simulink model "Eq_Zeq_denominator"  (R2022a)
settings: Solver=VariableStepAuto  StartTime=0.0  StopTime=10.0  RelTol=1e-3
settings Model: Creator=umber  LastModifiedBy=umber

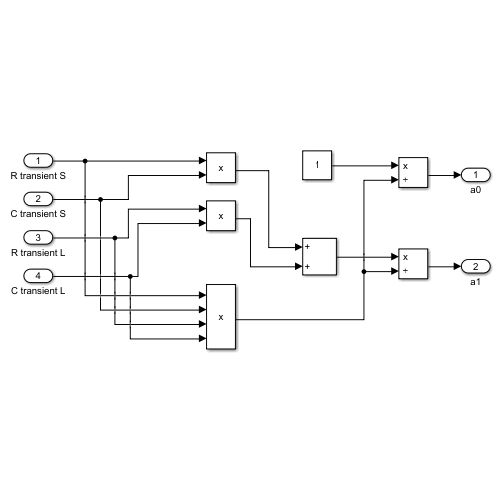
[thumbnail: Simulink's stored preview of the top-level diagram]
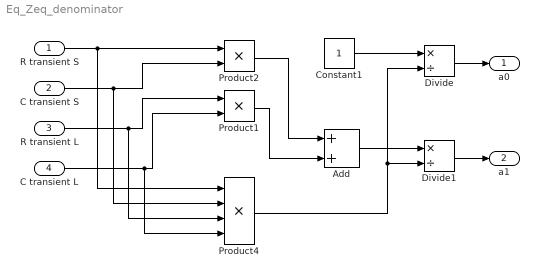
== system Eq_Zeq_denominator ==
  R transient S : Inport
  C transient S : Inport  Port=2
  R transient L : Inport  Port=3
  C transient L : Inport  Port=4
  Add : Sum
  Constant1 : Constant
  Divide : Product  Inputs=*/
  Divide1 : Product  Inputs=*/
  Product1 : Product
  Product2 : Product
  Product4 : Product  Inputs=4
  a0 : Outport
  a1 : Outport  Port=2
  wires:
  R transient S/1 -> Product4/1, Product2/1
  C transient S/1 -> Product4/2, Product2/2
  R transient L/1 -> Product4/3, Product1/1
  C transient L/1 -> Product4/4, Product1/2
  Product2/1 -> Add/1
  Product1/1 -> Add/2
  Add/1 -> Divide1/1
  Product4/1 -> Divide/2, Divide1/2
  Constant1/1 -> Divide/1
  Divide/1 -> a0/1
  Divide1/1 -> a1/1
